simulink model "model2"  (R2024b)
settings: Solver=ode4  StartTime=0.0  StopTime=20  FixedStep=1e-1  RelTol=1e-3
settings Model: Creator=Mehmet  LastModifiedBy=Mehmet

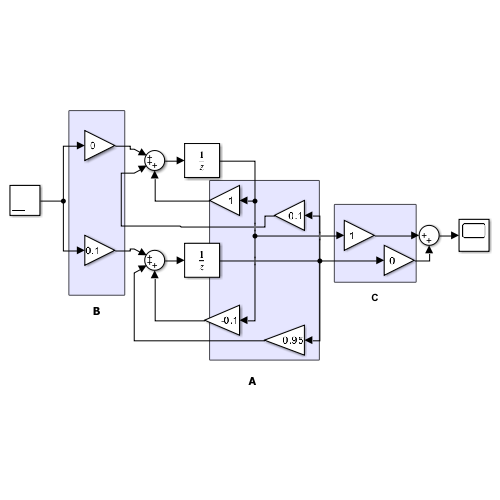
[thumbnail: Simulink's stored preview of the top-level diagram]
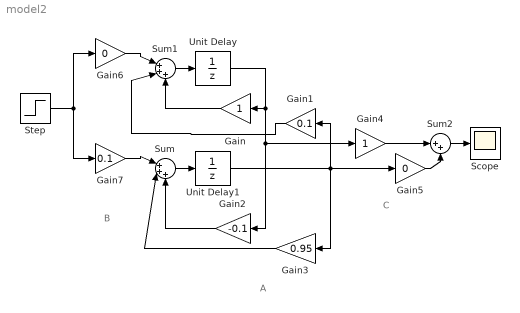
== system model2 ==
  note: C
  note: A
  note: B
  Gain : Gain
  Gain1 : Gain  Gain=0.1
  Gain2 : Gain  Gain=-0.1
  Gain3 : Gain  Gain=0.95
  Gain4 : Gain
  Gain5 : Gain  Gain=0
  Gain6 : Gain  Gain=0
  Gain7 : Gain  Gain=0.1
  Scope : Scope
  Step : Step  SampleTime=0
  Sum : Sum  Inputs=|+++
  Sum1 : Sum  Inputs=|+++
  Sum2 : Sum  Inputs=|++
  Unit Delay : UnitDelay  SampleTime=-1  HasFrameUpgradeWarning=on
  Unit Delay1 : UnitDelay  SampleTime=-1  HasFrameUpgradeWarning=on
  wires:
  Sum1/1 -> Unit Delay/1
  Sum/1 -> Unit Delay1/1
  Unit Delay/1 -> Gain4/1, Gain2/1, Gain/1
  Unit Delay1/1 -> Gain3/1, Gain5/1, Gain1/1
  Gain/1 -> Sum1/3
  Gain1/1 -> Sum1/2
  Gain2/1 -> Sum/3
  Gain3/1 -> Sum/2
  Gain4/1 -> Sum2/1
  Gain5/1 -> Sum2/2
  Gain6/1 -> Sum1/1
  Gain7/1 -> Sum/1
  Step/1 -> Gain7/1, Gain6/1
  Sum2/1 -> Scope/1
